simulink model "Quadrocopter"  (Simulink 8.6)
settings: Solver=ode5  StartTime=0.0  StopTime=Tsim  FixedStep=dT  MaxStep=0.01  RelTol=1e-3
settings Model: Creator=Kryzchu  LastModifiedBy=omera
settings DataIOCC: LimitDataPoints=off
settings DebuggingCC: FcnCallInpInsideContextMsg=EnableAllAsWarning
settings GRTTargetCC: CombineOutputUpdateFcns=on  GRTInterface=off

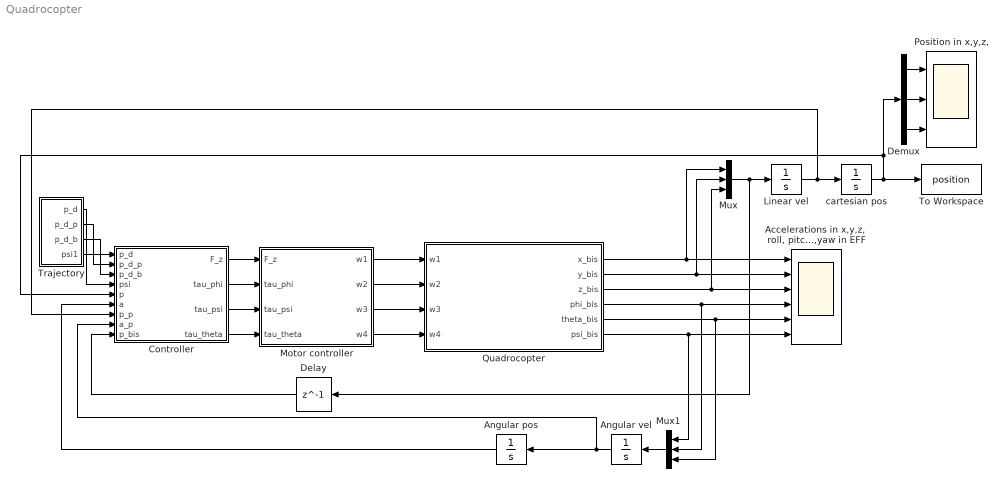
== system Quadrocopter ==
  "Accelerations in x,y,z,  roll, pitch,yaw in EFF" : Scope  NumInputPorts=6
  Angular pos : Integrator
  Angular vel : Integrator
  Controller : Subsystem
  Delay : Delay  DelayLength=1
  Demux : Demux  Outputs=3
  Linear vel : Integrator
  Motor controller : Subsystem
  Mux : Mux  Inputs=3
  Mux1 : Mux  Inputs=3
  "Position in x,y,z, " : Scope  NumInputPorts=3
  Quadrocopter : Subsystem
  To Workspace : ToWorkspace  VariableName=position  SampleTime=-1
  Trajectory : Subsystem
  cartesian pos : Integrator
  wires:
  Quadrocopter/1(x_bis) -> "Accelerations in x,y,z,  roll, pitch,yaw in EFF"/1, Mux/1
  Quadrocopter/2(y_bis) -> "Accelerations in x,y,z,  roll, pitch,yaw in EFF"/2, Mux/2
  Quadrocopter/3(z_bis) -> "Accelerations in x,y,z,  roll, pitch,yaw in EFF"/3, Mux/3
  Quadrocopter/4(phi_bis) -> "Accelerations in x,y,z,  roll, pitch,yaw in EFF"/4, Mux1/2
  Quadrocopter/5(theta_bis) -> "Accelerations in x,y,z,  roll, pitch,yaw in EFF"/5, Mux1/3
  Quadrocopter/6(psi_bis) -> "Accelerations in x,y,z,  roll, pitch,yaw in EFF"/6, Mux1/1
  Mux/1 -> Linear vel/1, Delay/1
  Linear vel/1 -> cartesian pos/1, Controller/7(p_p)
  cartesian pos/1 -> To Workspace/1, Demux/1, Controller/5(p)
  Motor controller/1(w1) -> Quadrocopter/1(w1)
  Motor controller/2(w2) -> Quadrocopter/2(w2)
  Motor controller/3(w3) -> Quadrocopter/3(w3)
  Motor controller/4(w4) -> Quadrocopter/4(w4)
  Controller/1(F_z) -> Motor controller/1(F_z)
  Controller/2(tau_phi) -> Motor controller/2(tau_phi)
  Controller/3(tau_psi) -> Motor controller/3(tau_psi)
  Controller/4(tau_theta) -> Motor controller/4(tau_theta)
  Mux1/1 -> Angular vel/1
  Angular vel/1 -> Angular pos/1, Controller/8(a_p)
  Angular pos/1 -> Controller/6(a)
  Trajectory/1(p_d) -> Controller/1(p_d)
  Demux/1 -> "Position in x,y,z, "/1
  Demux/2 -> "Position in x,y,z, "/2
  Demux/3 -> "Position in x,y,z, "/3
  Trajectory/4(psi1) -> Controller/4(psi)
  Delay/1 -> Controller/9(p_bis)
  Trajectory/2(p_d_p) -> Controller/2(p_d_p)
  Trajectory/3(p_d_b) -> Controller/3(p_d_b)

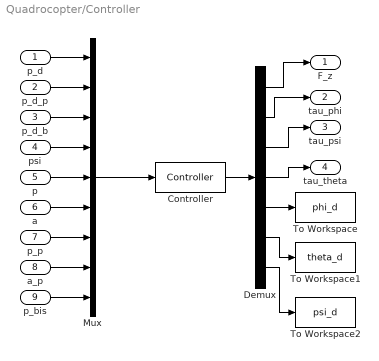
== system Quadrocopter/Controller ==
  p_d : Inport
  p_d_p : Inport  Port=2
  p_d_b : Inport  Port=3
  psi : Inport  Port=4
  p : Inport  Port=5
  a : Inport  Port=6
  p_p : Inport  Port=7
  a_p : Inport  Port=8
  p_bis : Inport  Port=9
  Controller : MATLABFcn  MATLABFcn=Controller  OutputDimensions=7
  Demux : Demux  Outputs=7
  Mux : Mux  Inputs=9
  To Workspace : ToWorkspace  VariableName=phi_d  SampleTime=-1
  To Workspace1 : ToWorkspace  VariableName=theta_d  SampleTime=-1
  To Workspace2 : ToWorkspace  VariableName=psi_d  SampleTime=-1
  F_z : Outport
  tau_phi : Outport  Port=2
  tau_psi : Outport  Port=3
  tau_theta : Outport  Port=4
  wires:
  p_d/1 -> Mux/1
  Mux/1 -> Controller/1
  Controller/1 -> Demux/1
  Demux/1 -> F_z/1
  Demux/2 -> tau_phi/1
  Demux/3 -> tau_psi/1
  Demux/4 -> tau_theta/1
  Demux/5 -> To Workspace/1
  Demux/6 -> To Workspace1/1
  Demux/7 -> To Workspace2/1
  p_d_p/1 -> Mux/2
  p_d_b/1 -> Mux/3
  psi/1 -> Mux/4
  p/1 -> Mux/5
  a/1 -> Mux/6
  p_p/1 -> Mux/7
  a_p/1 -> Mux/8
  p_bis/1 -> Mux/9

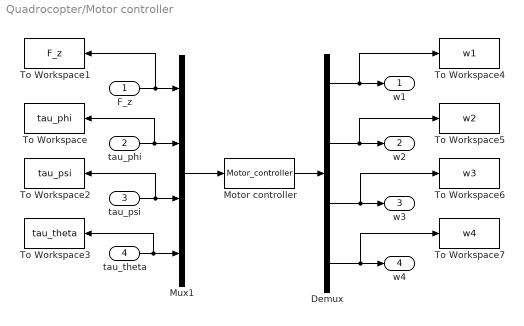
== system Quadrocopter/Motor controller ==
  F_z : Inport
  tau_phi : Inport  Port=2
  tau_psi : Inport  Port=3
  tau_theta : Inport  Port=4
  Demux : Demux
  Motor controller : MATLABFcn  MATLABFcn=Motor_controller  OutputDimensions=4
  Mux1 : Mux
  To Workspace : ToWorkspace  VariableName=tau_phi  SampleTime=-1
  To Workspace1 : ToWorkspace  VariableName=F_z  SampleTime=-1
  To Workspace2 : ToWorkspace  VariableName=tau_psi  SampleTime=-1
  To Workspace3 : ToWorkspace  VariableName=tau_theta  SampleTime=-1
  To Workspace4 : ToWorkspace  VariableName=w1  SampleTime=-1
  To Workspace5 : ToWorkspace  VariableName=w2  SampleTime=-1
  To Workspace6 : ToWorkspace  VariableName=w3  SampleTime=-1
  To Workspace7 : ToWorkspace  VariableName=w4  SampleTime=-1
  w1 : Outport
  w2 : Outport  Port=2
  w3 : Outport  Port=3
  w4 : Outport  Port=4
  wires:
  Motor controller/1 -> Demux/1
  F_z/1 -> To Workspace1/1, Mux1/1
  Demux/1 -> To Workspace4/1, w1/1
  tau_phi/1 -> To Workspace/1, Mux1/2
  Demux/3 -> To Workspace6/1, w3/1
  tau_psi/1 -> To Workspace2/1, Mux1/3
  Demux/4 -> To Workspace7/1, w4/1
  tau_theta/1 -> To Workspace3/1, Mux1/4
  Mux1/1 -> Motor controller/1
  Demux/2 -> To Workspace5/1, w2/1

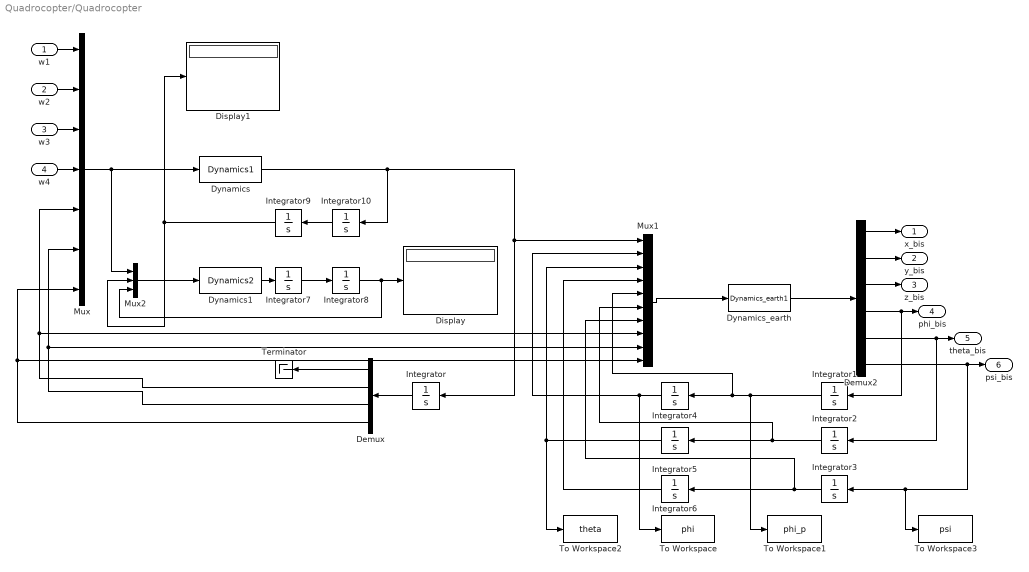
== system Quadrocopter/Quadrocopter ==
  w1 : Inport
  w2 : Inport  Port=2
  w3 : Inport  Port=3
  w4 : Inport  Port=4
  Demux : Demux
  Demux2 : Demux  Outputs=6
  Display : Display
      settings: Decimation=4
  Display1 : Display
      settings: Decimation=4
  Dynamics : MATLABFcn  MATLABFcn=Dynamics1  OutputDimensions=4
  Dynamics1 : MATLABFcn  MATLABFcn=Dynamics2  OutputDimensions=4
  Dynamics_earth : MATLABFcn  MATLABFcn=Dynamics_earth1  OutputDimensions=6
  Integrator{,1..10} (11 alike) : Integrator
  Mux : Mux  Inputs=7
  Mux1 : Mux  Inputs=10
  Mux2 : Mux  Inputs=3
  Terminator : Terminator
  To Workspace : ToWorkspace  VariableName=phi  SampleTime=-1
  To Workspace1 : ToWorkspace  VariableName=phi_p  SampleTime=-1
  To Workspace2 : ToWorkspace  VariableName=theta  SampleTime=-1
  To Workspace3 : ToWorkspace  VariableName=psi  SampleTime=-1
  x_bis : Outport
  y_bis : Outport  Port=2
  z_bis : Outport  Port=3
  phi_bis : Outport  Port=4
  theta_bis : Outport  Port=5
  psi_bis : Outport  Port=6
  wires:
  Mux/1 -> Mux2/1, Dynamics/1
  Dynamics/1 -> Integrator10/1, Integrator/1, Mux1/1
  Integrator/1 -> Demux/1
  Demux/4 -> Mux/7, Mux1/10
  Demux/3 -> Mux/6, Mux1/9
  Demux/2 -> Mux/5, Mux1/8
  Mux1/1 -> Dynamics_earth/1
  Dynamics_earth/1 -> Demux2/1
  Demux2/4 -> phi_bis/1, Integrator1/1
  Demux2/5 -> theta_bis/1, Integrator2/1
  Demux2/6 -> psi_bis/1, Integrator3/1, To Workspace3/1
  Integrator1/1 -> Integrator4/1, Mux1/5, To Workspace1/1
  Integrator2/1 -> Integrator5/1, Mux1/6
  Integrator3/1 -> Integrator6/1, Mux1/7
  Integrator4/1 -> Mux1/2, To Workspace/1
  Integrator5/1 -> Mux1/3, To Workspace2/1
  Integrator6/1 -> Mux1/4
  w1/1 -> Mux/1
  w2/1 -> Mux/2
  w3/1 -> Mux/3
  w4/1 -> Mux/4
  Demux2/1 -> x_bis/1
  Demux2/2 -> y_bis/1
  Demux2/3 -> z_bis/1
  Demux/1 -> Terminator/1
  Integrator7/1 -> Integrator8/1
  Dynamics1/1 -> Integrator7/1
  Mux2/1 -> Dynamics1/1
  Integrator8/1 -> Mux2/3, Display/1
  Integrator10/1 -> Integrator9/1
  Integrator9/1 -> Mux2/2, Display1/1

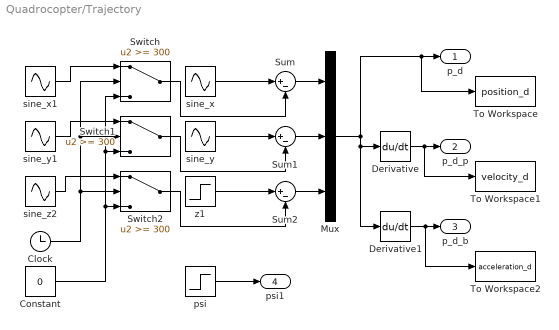
== system Quadrocopter/Trajectory ==
  Clock : Clock
  Constant : Constant  Value=0
  Derivative : Derivative
  Derivative1 : Derivative
  Mux : Mux  Inputs=3
  Sum : Sum  Inputs=|+-
  Sum1 : Sum  Inputs=|+-
  Sum2 : Sum  Inputs=|+-
  Switch : Switch  Threshold=300
  Switch1 : Switch  Threshold=300
  Switch2 : Switch  Threshold=300
  To Workspace : ToWorkspace  VariableName=position_d  SampleTime=-1
  To Workspace1 : ToWorkspace  VariableName=velocity_d  SampleTime=-1
  To Workspace2 : ToWorkspace  VariableName=acceleration_d  SampleTime=-1
  psi : Step  Time=0  After=0  SampleTime=0  ZeroCross=off
  sine_x : Sin  Amplitude=2  Frequency=0.04  SampleTime=0
  sine_x1 : Sin  Frequency=0.04  SampleTime=0
  sine_y : Sin  Amplitude=2  Frequency=0.04  Phase=pi/2  SampleTime=0
  sine_y1 : Sin  Frequency=0.04  Phase=pi/2  SampleTime=0
  sine_z2 : Sin  Frequency=0.4  Phase=pi/2  SampleTime=0
  z1 : Step  Time=150  After=2  SampleTime=0  ZeroCross=off
  p_d : Outport
  p_d_p : Outport  Port=2
  p_d_b : Outport  Port=3
  psi1 : Outport  Port=4
  wires:
  psi/1 -> psi1/1
  Mux/1 -> To Workspace/1, p_d/1, Derivative1/1, Derivative/1
  Sum/1 -> Mux/1
  Sum1/1 -> Mux/2
  Sum2/1 -> Mux/3
  Clock/1 -> Switch2/2, Switch1/2, Switch/2
  Switch/1 -> Sum/2
  Switch1/1 -> Sum1/2
  Switch2/1 -> Sum2/2
  sine_x1/1 -> Switch/1
  sine_y1/1 -> Switch1/1
  Constant/1 -> Switch2/3, Switch/3, Switch1/3
  sine_z2/1 -> Switch2/1
  z1/1 -> Sum2/1
  Derivative/1 -> To Workspace1/1, p_d_p/1
  Derivative1/1 -> To Workspace2/1, p_d_b/1
  sine_x/1 -> Sum/1
  sine_y/1 -> Sum1/1
